simulink model "planGlobal_simfcn"  (R2024b)
settings: Solver=VariableStepAuto  StartTime=0.0  StopTime=10.0  RelTol=1e-3
InitFcn:
  | globalPlanSetup
undefined symbols (not defined in the file): dem, goal, gridLoc, start, tuneableTerrainAwareParams, worldRes
libraries: roshelperlib x2
settings Model: Creator=cstabile  LastModifiedBy=jbrault
settings SolverCC: DateTimeAtSimulationTimeZero=[]

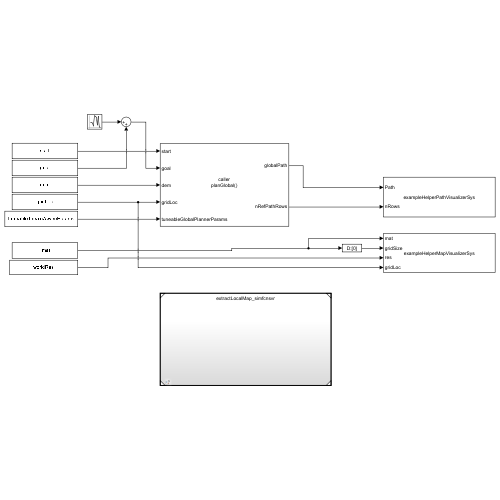
[thumbnail: Simulink's stored preview of the top-level diagram]
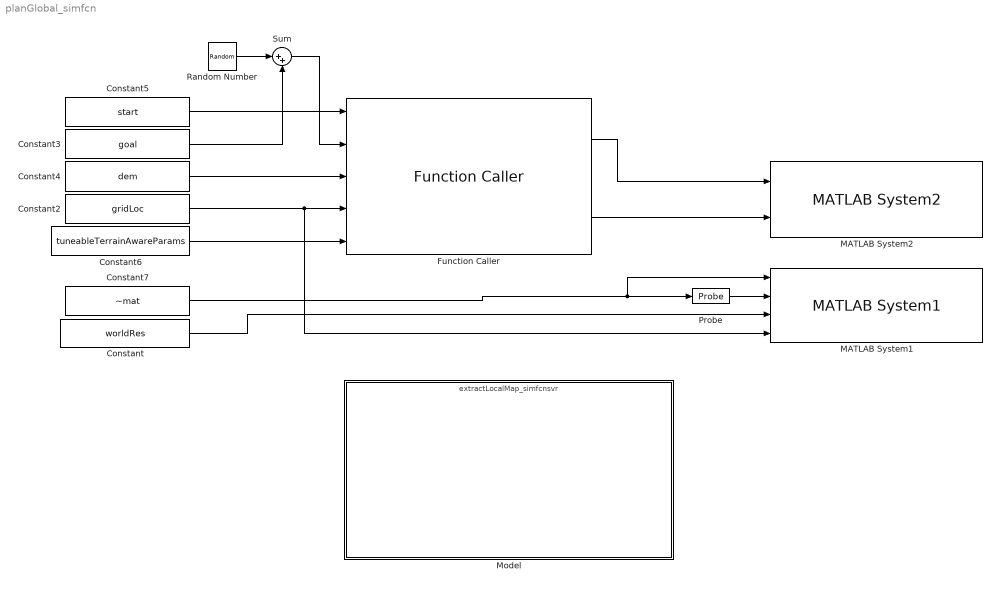
== system planGlobal_simfcn ==
  Constant : Constant  Value=worldRes
  Constant2 : Constant  Value=gridLoc
  Constant3 : Constant  Value=goal
  Constant4 : Constant  Value=dem
  Constant5 : Constant  Value=start
  Constant6 : Constant  Value=tuneableTerrainAwareParams  OutDataTypeStr=Bus: fsp_tunable_bus
  Constant7 : Constant  Value=~mat
  Function Caller : FunctionCaller  FunctionPrototype=[globalPath,nRefPathRows] = planGlobal(start,goal,dem,gridLoc,tuneableGlobalPlannerParams)  InputArgumentSpecifications=<Enter example>  OutputArgumentSpecifications=<Enter example>
  MATLAB System1 : roshelperlib/MATLAB System1  MapType=SDF  IsEgo=off  DisplayVisual=on  SimulateUsing=Interpreted execution
  MATLAB System2 : roshelperlib/MATLAB System2  VisualizationParameters={'k-'}  PlotType=Line  DisplayVisual=on  SimulateUsing=Interpreted execution
  Model : ModelReference  ModelNameDialog=extractLocalMap_simfcnsvr.slx  SimulationMode=Normal  ScheduleRates=on  ModelReferenceVersion=2.0
  Probe : Probe  ProbeWidth=off  ProbeSampleTime=off  ProbeComplexSignal=off  ProbeSignalDimensions=on
  Random Number : RandomNumber  Mean=[0 0 0]  Variance=10  SampleTime=0.1
  Sum : Sum  Inputs=|++
  wires:
  Constant2/1 -> MATLAB System1/4, Function Caller/4
  Constant4/1 -> Function Caller/3
  Constant5/1 -> Function Caller/1
  Constant3/1 -> Sum/2
  Constant6/1 -> Function Caller/5
  Function Caller/1 -> MATLAB System2/1
  Function Caller/2 -> MATLAB System2/2
  Constant/1 -> MATLAB System1/3
  Probe/1 -> MATLAB System1/2
  Random Number/1 -> Sum/1
  Sum/1 -> Function Caller/2
  Constant7/1 -> MATLAB System1/1, Probe/1
